simulink model "HDL_AXI"  (R2020a)
settings: Solver=FixedStepDiscrete  StartTime=0.0  StopTime=length(stream_in)  RelTol=1e-3
PreLoadFcn:
  | video_filename = 'vipmen.avi';
  | 
  | v = VideoReader(video_filename);
  | frame_height = v.Height;
  | frame_width = v.Width;
  | save video_handle v
  | 
  | stream_in = zeros(ceil(v.FrameRate*v.Duration*v.Height*v.Width),1);
  | 
  | i = 1;
  | while hasFrame(v)
  |     frame = rgb2gray(readFrame(v));
  |     a = reshape(frame',[],1);
  |     stream_in(i:i+length(a)-1) = a;
  |     i = i + length(a);
  | end
  | 
  | save stream_in stream_in
InitFcn:
  | load stream_in;
StopFcn:
  | save stream_out stream_out;
libraries: xbsIndex_r4 x11, dspsrcs4 x1
settings Model: Creator=abehbood  LastModifiedBy=viswanad
settings DataIOCC: ReturnWorkspaceOutputs=off
settings OptimizationCC: LifeSpan=inf
settings DebuggingCC: SFExecutionAtInitializationDiag=none  ArithmeticOperatorsInVariantConditions=warning
settings SFSimCC: SimUseLocalCustomCode=off  CustomCodeUndefinedFunction=UseInterfaceOnly
settings RTWCC: RTWUseLocalCustomCode=off
settings CodeAppCC: StateflowObjectComments=on

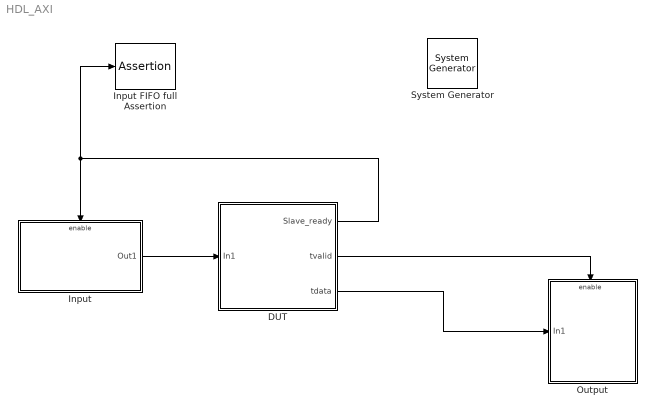
== system HDL_AXI ==
  " System Generator" : xbsIndex_r4/ System Generator  Tag=genX  xilinxfamily=kintex7  part=xc7k325t  speed=-3  package=fbg676  synthesis_tool=Vivado  clock_wrapper=Clock Enables  directory=./netlist  proj_type=Vivado  Synth_file=Vivado Synthesis Defaults  Impl_file=Vivado Implementation Defaults  testbench=on  simulink_period=1  sysclk_period=10  dcm_input_clock_period=10  incr_netlist=off  trim_vbits=Everywhere in SubSystem  dbl_ovrd=According to Block Masks  core_generation=According to Block Masks  run_coregen=off  deprecated_control=off  eval_field=0  block_type=sysgen
  DUT : Subsystem
  Input : Subsystem
  Input FIFO full Assertion : Assertion  Enabled=off  AssertionFailFcn=warning('Input buffer full.')  StopWhenAssertionFail=off
  Output : Subsystem
  wires:
  DUT/3(tdata) -> Output/1(In1)
  Input/1(Out1) -> DUT/1(In1)
  DUT/1("Slave_ready ") -> Input FIFO full Assertion/1, Input/Enable
  DUT/2(tvalid) -> Output/Enable

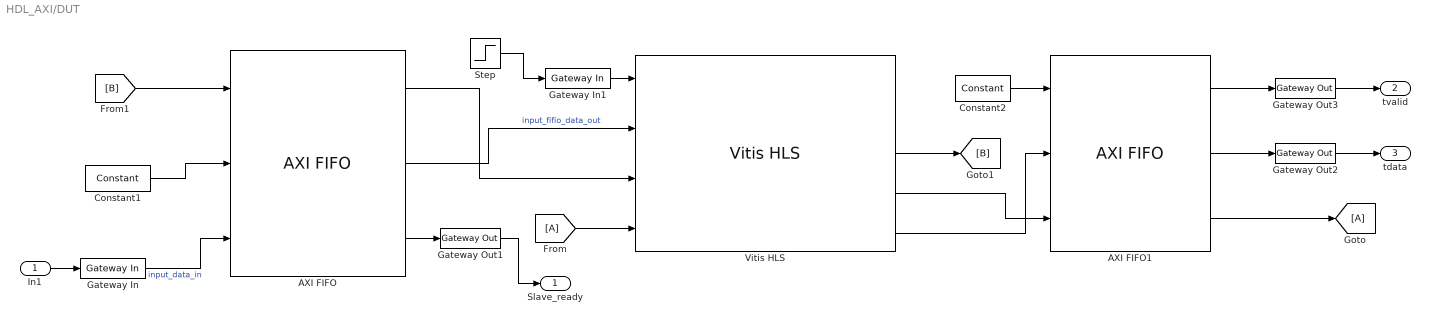
== system HDL_AXI/DUT ==
  In1 : Inport
  AXI FIFO : xbsIndex_r4/AXI FIFO  input_depth_axis=1K  actual_fifo_depth_label=1026  enable_tdata=on  enable_tdest=off  enable_tstrb=off  enable_tready=on  enable_tid=off  enable_tuser=off  enable_tkeep=off  enable_tlast=off  has_aresetn=off  enable_data_counts_axis=off  fifo_implementation_type_axis=Common Clock Block RAM  trim_axipin_name=off  programmable_full_type_axis=Full  full_threshold_assert_value_axis=0  programmable_empty_type_axis=Empty  empty_threshold_assert_value_axis=1022  underflow_flag_axi=0  underflow_sense_axi=Active High  overflow_flag_axi=0  overflow_sense_axi=Active High  simulation_type=fast_sim  block_type=axi_fifo
  AXI FIFO1 : xbsIndex_r4/AXI FIFO  input_depth_axis=1K  actual_fifo_depth_label=1026  enable_tdata=on  enable_tdest=off  enable_tstrb=off  enable_tready=on  enable_tid=off  enable_tuser=off  enable_tkeep=off  enable_tlast=off  has_aresetn=off  enable_data_counts_axis=off  fifo_implementation_type_axis=Common Clock Block RAM  trim_axipin_name=off  programmable_full_type_axis=Full  full_threshold_assert_value_axis=0  programmable_empty_type_axis=Empty  empty_threshold_assert_value_axis=1022  underflow_flag_axi=0  underflow_sense_axi=Active High  overflow_flag_axi=0  overflow_sense_axi=Active High  simulation_type=fast_sim  block_type=axi_fifo
  Constant1 : xbsIndex_r4/Constant  const=1  gui_display_data_type=Boolean  arith_type=Boolean  n_bits=16  bin_pt=14  preci_type=Single  exp_width=8  frac_width=24  explicit_period=on  period=1  equ=P=C  opselect=C  inp2=PCIN>>17  opr=+  inp1=P  carry=CIN  dbl_ovrd=off  block_type=constant
  Constant2 : xbsIndex_r4/Constant  const=1  gui_display_data_type=Boolean  arith_type=Boolean  n_bits=16  bin_pt=14  preci_type=Single  exp_width=8  frac_width=24  explicit_period=on  period=1  equ=P=C  opselect=C  inp2=PCIN>>17  opr=+  inp1=P  carry=CIN  dbl_ovrd=off  block_type=constant
  Gateway In : xbsIndex_r4/Gateway In  gui_display_data_type=Fixed-point  arith_type=Unsigned  n_bits=8  bin_pt=0  preci_type=Single  exp_width=8  frac_width=24  rows=1  columns=1  quantization="Round  (unbiased: +/- Inf)"  overflow=Saturate  period=1  UseAsADC=off  ADCChannel='1'  interface=None  automatic_assignment=on  address_offset=hex2dec('00')  intf_name=''  intf_description=''  default_value=0  timing_constraint=None  locs_specified=off  LOCs={}  io_standard={}  inherit_from_input=off  hdl_port=on  dbl_ovrd=off  block_type=gatewayin
  Gateway In1 : xbsIndex_r4/Gateway In  gui_display_data_type=Boolean  arith_type=Boolean  n_bits=16  bin_pt=14  preci_type=Single  exp_width=8  frac_width=24  rows=1  columns=1  quantization="Round  (unbiased: +/- Inf)"  overflow=Saturate  period=1  UseAsADC=off  ADCChannel='1'  interface=None  automatic_assignment=on  address_offset=hex2dec('00')  intf_name=''  intf_description=''  default_value=0  timing_constraint=None  locs_specified=off  LOCs={}  io_standard={}  inherit_from_input=off  hdl_port=on  dbl_ovrd=off  block_type=gatewayin
  Gateway Out1 : xbsIndex_r4/Gateway Out  inherit_from_input=off  hdl_port=on  rows=1  columns=1  UseAsDAC=off  DACChannel='1'  interface=None  automatic_assignment=on  address_offset=hex2dec('00')  intf_name=''  intf_description=''  timing_constraint=None  locs_specified=off  LOCs={}  io_standard={}  block_type=gatewayout
  Gateway Out2 : xbsIndex_r4/Gateway Out  inherit_from_input=on  hdl_port=on  rows=1  columns=1  UseAsDAC=off  DACChannel='1'  interface=None  automatic_assignment=on  address_offset=hex2dec('00')  intf_name=''  intf_description=''  timing_constraint=None  locs_specified=off  LOCs={}  io_standard={}  block_type=gatewayout
  Gateway Out3 : xbsIndex_r4/Gateway Out  inherit_from_input=on  hdl_port=on  rows=1  columns=1  UseAsDAC=off  DACChannel='1'  interface=None  automatic_assignment=on  address_offset=hex2dec('00')  intf_name=''  intf_description=''  timing_constraint=None  locs_specified=off  LOCs={}  io_standard={}  block_type=gatewayout
  Step : Step  Time=2  SampleTime=1
  Vitis HLS : xbsIndex_r4/Vitis HLS  anytable='./code_HLS/ModelComposerDesign_prj/solution1'  fast_sim=off  display_datatype=off  rate_propagation_method=Simulink system period  model_file_path=''  latency=1  block_type=vitis_hls
      settings: infoedit=This block allows including C,C++ and SystemC source files in System Generator for DSP designs.
  "Slave_ready " : Outport
  tvalid : Outport  Port=2
  tdata : Outport  Port=3
  wires:
  In1/1 -> Gateway In/1
  Gateway In/1 -> AXI FIFO/3  "input_data_in"
  AXI FIFO/3 -> Gateway Out1/1
  Constant1/1 -> AXI FIFO/2
  Gateway Out1/1 -> "Slave_ready "/1
  [B] -> AXI FIFO/1
  AXI FIFO1/1 -> Gateway Out3/1
  AXI FIFO1/2 -> Gateway Out2/1
  Gateway Out2/1 -> tdata/1
  AXI FIFO1/3 -> [A]
  Constant2/1 -> AXI FIFO1/1
  Gateway Out3/1 -> tvalid/1
  Step/1 -> Gateway In1/1
  [A] -> Vitis HLS/4
  Vitis HLS/4 -> AXI FIFO1/3
  AXI FIFO/2 -> Vitis HLS/2  "input_fifio_data_out"
  AXI FIFO/1 -> Vitis HLS/3
  Vitis HLS/3 -> [B]
  Gateway In1/1 -> Vitis HLS/1
  Vitis HLS/5 -> AXI FIFO1/2

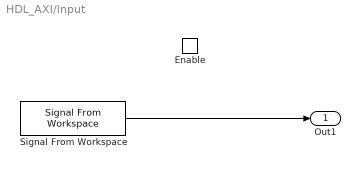
== system HDL_AXI/Input ==
  Enable : EnablePort
  Signal From Workspace : dspsrcs4/Signal From Workspace  X=stream_in  Ts=1  nsamps=1  OutputAfterFinalValue=Setting to zero  ignoreOrWarnInputAndFrameLengths=off  OutputFrames=off
  Out1 : Outport
  wires:
  Signal From Workspace/1 -> Out1/1

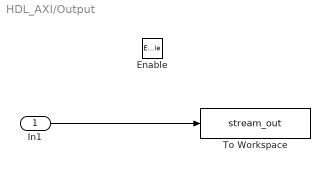
== system HDL_AXI/Output ==
  In1 : Inport
  Enable : EnablePort
  To Workspace : ToWorkspace  VariableName=stream_out  SampleTime=-1
  wires:
  In1/1 -> To Workspace/1
